simulink model "sampleModel1488"  (R2023a)
settings: Solver=VariableStepAuto  StartTime=0.0  StopTime=10.0  RelTol=1e-3
undefined symbols (not defined in the file): b011101a, b0c8, bf87616c, DiscIntNeverNeededParam, Newton, Raphson
libraries: simulink x171, slpidlib x32, simulink_need_slupdate x2
(part 3 of 6)

== system sampleModel1488/cfblk129/cfblk7 ==
  cfblk1 : Inport
  cfblk14 : Inport  Port=2
  cfblk15 : Inport  Port=3
  cfblk10 : Product  Inputs=**
  cfblk11 : Sum  Inputs=+-
  cfblk12 : Signum
  cfblk13 : Bias  Bias=[839960934.882999]  SaturateOnIntegerOverflow=off
  cfblk16 : Delay  SampleTime=1
  cfblk17 : Delay  SampleTime=1
  cfblk3 : slpidlib/PID Controller  Controller=PID  Form=Parallel  TimeDomain=Discrete-time  UseExternalTs=off  SampleTime=1  IntegratorMethod=Forward Euler  FilterMethod=Forward Euler  ControllerParametersSource=internal  P=1  I=1  UseKiTs=off  D=0  N=100  UseFilter=on  TunerSelectOption=Transfer Function Based (PID Tuner App)  InitialConditionSource=internal  InitialConditionForIntegrator=0  InitialConditionForFilter=0  DifferentiatorICPrevScaledInput=0  ExternalReset=none  TrackingMode=off  Kt=1  LimitOutput=off  SatLimitsSource=internal  UpperSaturationLimit=inf  LowerSaturationLimit=-inf  LinearizeAsGain=off  AntiWindupMode=none  Kb=1  LimitIntegrator=off  UpperIntegratorSaturationLimit=inf  LowerIntegratorSaturationLimit=-inf  POutMin=[]  POutMax=[]  IOutMin=[]  IOutMax=[]  DOutMin=[]  DOutMax=[]  NOutMin=[]  NOutMax=[]  SumOutMin=[]  SumOutMax=[]  SaturationOutMin=[]  SaturationOutMax=[]  PParamMin=[]  PParamMax=[]  IParamMin=[]  IParamMax=[]  DParamMin=[]  DParamMax=[]  NParamMin=[]  NParamMax=[]  KbParamMin=[]  KbParamMax=[]  KtParamMin=[]  KtParamMax=[]  KbOutMin=[]  KbOutMax=[]  KtOutMin=[]  KtOutMax=[]  IntegratorOutMin=[]  IntegratorOutMax=[]  FilterOutMin=[]  FilterOutMax=[]  SumI1OutMin=[]  SumI1OutMax=[]  SumI2OutMin=[]  SumI2OutMax=[]  SumI3OutMin=[]  SumI3OutMax=[]  SumI4OutMin=[]  SumI4OutMax=[]  SumDOutMin=[]  SumDOutMax=[]  DifferentiatorOutMin=[]  DifferentiatorOutMax=[]  FilterDiffOutCoefMin=[]  FilterDiffOutCoefMax=[]  ReciprocalOutMin=[]  ReciprocalOutMax=[]  SumDenOutMin=[]  SumDenOutMax=[]  SumNumOutMin=[]  SumNumOutMax=[]  DivideOutMin=[]  DivideOutMax=[]  UdiffTsProdOutMin=[]  UdiffTsProdOutMax=[]  NTsProdOutMin=[]  NTsProdOutMax=[]  UintegralTsProdOutMin=[]  UintegralTsProdOutMax=[]  UngainTsProdOutMin=[]  UngainTsProdOutMax=[]  ClampingZeroOutDataTypeStr=Inherit: Inherit via back propagation  ClampingZeroOutMin=[]  ClampingZeroOutMax=[]  FilterDenConstantOutDataTypeStr=Inherit: Inherit via back propagation  FilterDenConstantOutMin=[]  FilterDenConstantOutMax=[]  PCopyOutDataTypeStr=Inherit: Inherit via back propagation  PCopyOutMin=[]  PCopyOutMax=[]  NCopyOutDataTypeStr=Inherit: Inherit via back propagation  NCopyOutMin=[]  NCopyOutMax=[]  IntegratorContinuousStateAttributes=''  IntegratorStateMustResolveToSignalObject=off  IntegratorRTWStateStorageClass=Auto  FilterContinuousStateAttributes=''  FilterStateMustResolveToSignalObject=off  FilterRTWStateStorageClass=Auto  ParallelPVariant=InternalParameters  IdealPVariant=Disabled  IVariant=InternalParameters  DVariant=InternalParameters  IntegratorVariant=Discrete  SatVariant=Disabled  AWVariant=Passthrough  PCopyVariant=Disabled  TRVariant=Disabled  FdbkBlocksVariant=Forward  IdealPFdbkVariant=Disabled  SatFdbkVariant=Disabled  DerivativeFilterVariant=ForwardEulerFilter  NVariant=InternalParameters  NCopyVariant=Disabled  FilterICVariant=InternalICsFilter  IntegratorICVariant=InternalICs  ExternalResetVariant=Disabled  TRSumVariant=Passthrough  SumFdbkVariant=Disabled  SumVariant=Sum_PID  TsampFilterVariant=InternalTs  TsampNgainVariant=Passthrough  TsampIntegralVariant=Disabled_SignalSpec  ExternalSaturationOutDataTypeStr=Inherit: Same as second input
      settings: LibrarySourceBlock=simulink/Discrete/Discrete PID Controller
  cfblk4 : DiscreteFir  SampleTime=1
  cfblk5 : slpidlib/PID Controller  Controller=PID  Form=Parallel  TimeDomain=Discrete-time  UseExternalTs=off  SampleTime=1  IntegratorMethod=Forward Euler  FilterMethod=Forward Euler  ControllerParametersSource=internal  P=1  I=1  UseKiTs=off  D=0  N=100  UseFilter=on  TunerSelectOption=Transfer Function Based (PID Tuner App)  InitialConditionSource=internal  InitialConditionForIntegrator=0  InitialConditionForFilter=0  DifferentiatorICPrevScaledInput=0  ExternalReset=none  TrackingMode=off  Kt=1  LimitOutput=off  SatLimitsSource=internal  UpperSaturationLimit=inf  LowerSaturationLimit=-inf  LinearizeAsGain=off  AntiWindupMode=none  Kb=1  LimitIntegrator=off  UpperIntegratorSaturationLimit=inf  LowerIntegratorSaturationLimit=-inf  POutMin=[]  POutMax=[]  IOutMin=[]  IOutMax=[]  DOutMin=[]  DOutMax=[]  NOutMin=[]  NOutMax=[]  SumOutMin=[]  SumOutMax=[]  SaturationOutMin=[]  SaturationOutMax=[]  PParamMin=[]  PParamMax=[]  IParamMin=[]  IParamMax=[]  DParamMin=[]  DParamMax=[]  NParamMin=[]  NParamMax=[]  KbParamMin=[]  KbParamMax=[]  KtParamMin=[]  KtParamMax=[]  KbOutMin=[]  KbOutMax=[]  KtOutMin=[]  KtOutMax=[]  IntegratorOutMin=[]  IntegratorOutMax=[]  FilterOutMin=[]  FilterOutMax=[]  SumI1OutMin=[]  SumI1OutMax=[]  SumI2OutMin=[]  SumI2OutMax=[]  SumI3OutMin=[]  SumI3OutMax=[]  SumI4OutMin=[]  SumI4OutMax=[]  SumDOutMin=[]  SumDOutMax=[]  DifferentiatorOutMin=[]  DifferentiatorOutMax=[]  FilterDiffOutCoefMin=[]  FilterDiffOutCoefMax=[]  ReciprocalOutMin=[]  ReciprocalOutMax=[]  SumDenOutMin=[]  SumDenOutMax=[]  SumNumOutMin=[]  SumNumOutMax=[]  DivideOutMin=[]  DivideOutMax=[]  UdiffTsProdOutMin=[]  UdiffTsProdOutMax=[]  NTsProdOutMin=[]  NTsProdOutMax=[]  UintegralTsProdOutMin=[]  UintegralTsProdOutMax=[]  UngainTsProdOutMin=[]  UngainTsProdOutMax=[]  ClampingZeroOutDataTypeStr=Inherit: Inherit via back propagation  ClampingZeroOutMin=[]  ClampingZeroOutMax=[]  FilterDenConstantOutDataTypeStr=Inherit: Inherit via back propagation  FilterDenConstantOutMin=[]  FilterDenConstantOutMax=[]  PCopyOutDataTypeStr=Inherit: Inherit via back propagation  PCopyOutMin=[]  PCopyOutMax=[]  NCopyOutDataTypeStr=Inherit: Inherit via back propagation  NCopyOutMin=[]  NCopyOutMax=[]  IntegratorContinuousStateAttributes=''  IntegratorStateMustResolveToSignalObject=off  IntegratorRTWStateStorageClass=Auto  FilterContinuousStateAttributes=''  FilterStateMustResolveToSignalObject=off  FilterRTWStateStorageClass=Auto  ParallelPVariant=InternalParameters  IdealPVariant=Disabled  IVariant=InternalParameters  DVariant=InternalParameters  IntegratorVariant=Discrete  SatVariant=Disabled  AWVariant=Passthrough  PCopyVariant=Disabled  TRVariant=Disabled  FdbkBlocksVariant=Forward  IdealPFdbkVariant=Disabled  SatFdbkVariant=Disabled  DerivativeFilterVariant=ForwardEulerFilter  NVariant=InternalParameters  NCopyVariant=Disabled  FilterICVariant=InternalICsFilter  IntegratorICVariant=InternalICs  ExternalResetVariant=Disabled  TRSumVariant=Passthrough  SumFdbkVariant=Disabled  SumVariant=Sum_PID  TsampFilterVariant=InternalTs  TsampNgainVariant=Passthrough  TsampIntegralVariant=Disabled_SignalSpec  ExternalSaturationOutDataTypeStr=Inherit: Same as second input
      settings: LibrarySourceBlock=simulink/Discrete/Discrete PID Controller
  cfblk6 : simulink/Discrete/Difference  ICPrevInput=0.0  OutMin=[]  OutMax=[]  OutDataTypeStr=Inherit: Inherit via back propagation  OutDataType=fixdt(1, 16)  OutScaling=2^-10  DoSatur=off
  cfblk7 : slpidlib/PID Controller (2DOF)  Controller=PID  Form=Parallel  TimeDomain=Discrete-time  UseExternalTs=off  SampleTime=1  IntegratorMethod=Forward Euler  FilterMethod=Forward Euler  ControllerParametersSource=internal  P=1  I=1  UseKiTs=off  D=0  N=100  UseFilter=on  b=1  c=1  TunerSelectOption=Transfer Function Based (PID Tuner App)  InitialConditionSource=internal  InitialConditionForIntegrator=0  InitialConditionForFilter=0  DifferentiatorICPrevScaledInput=0  ExternalReset=none  TrackingMode=off  Kt=1  LimitOutput=off  SatLimitsSource=internal  UpperSaturationLimit=inf  LowerSaturationLimit=-inf  LinearizeAsGain=off  AntiWindupMode=none  Kb=1  LimitIntegrator=off  UpperIntegratorSaturationLimit=inf  LowerIntegratorSaturationLimit=-inf  POutMin=[]  POutMax=[]  IOutMin=[]  IOutMax=[]  DOutMin=[]  DOutMax=[]  NOutMin=[]  NOutMax=[]  bOutMin=[]  bOutMax=[]  cOutMin=[]  cOutMax=[]  SumOutMin=[]  SumOutMax=[]  SaturationOutMin=[]  SaturationOutMax=[]  PParamMin=[]  PParamMax=[]  IParamMin=[]  IParamMax=[]  DParamMin=[]  DParamMax=[]  NParamMin=[]  NParamMax=[]  bParamMin=[]  bParamMax=[]  cParamMin=[]  cParamMax=[]  KbParamMin=[]  KbParamMax=[]  KtParamMin=[]  KtParamMax=[]  KbOutMin=[]  KbOutMax=[]  KtOutMin=[]  KtOutMax=[]  IntegratorOutMin=[]  IntegratorOutMax=[]  FilterOutMin=[]  FilterOutMax=[]  SumI1OutMin=[]  SumI1OutMax=[]  SumI2OutMin=[]  SumI2OutMax=[]  SumI3OutMin=[]  SumI3OutMax=[]  SumI4OutMin=[]  SumI4OutMax=[]  SumDOutMin=[]  SumDOutMax=[]  Sum1OutMin=[]  Sum1OutMax=[]  Sum2OutMin=[]  Sum2OutMax=[]  Sum3OutMin=[]  Sum3OutMax=[]  DifferentiatorOutMin=[]  DifferentiatorOutMax=[]  FilterDiffOutCoefMin=[]  FilterDiffOutCoefMax=[]  ReciprocalOutMin=[]  ReciprocalOutMax=[]  SumDenOutMin=[]  SumDenOutMax=[]  SumNumOutMin=[]  SumNumOutMax=[]  DivideOutMin=[]  DivideOutMax=[]  UdiffTsProdOutMin=[]  UdiffTsProdOutMax=[]  NTsProdOutMin=[]  NTsProdOutMax=[]  UintegralTsProdOutMin=[]  UintegralTsProdOutMax=[]  UngainTsProdOutMin=[]  UngainTsProdOutMax=[]  ClampingZeroOutDataTypeStr=Inherit: Inherit via back propagation  ClampingZeroOutMin=[]  ClampingZeroOutMax=[]  FilterDenConstantOutDataTypeStr=Inherit: Inherit via back propagation  FilterDenConstantOutMin=[]  FilterDenConstantOutMax=[]  PCopyOutDataTypeStr=Inherit: Inherit via back propagation  PCopyOutMin=[]  PCopyOutMax=[]  NCopyOutDataTypeStr=Inherit: Inherit via back propagation  NCopyOutMin=[]  NCopyOutMax=[]  IntegratorContinuousStateAttributes=''  IntegratorStateMustResolveToSignalObject=off  IntegratorRTWStateStorageClass=Auto  FilterContinuousStateAttributes=''  FilterStateMustResolveToSignalObject=off  FilterRTWStateStorageClass=Auto  ParallelPVariant=InternalParameters  IdealPVariant=Disabled  IVariant=InternalParameters  DVariant=InternalParameters  bVariant=InternalParameters  cVariant=InternalParameters  IntegratorVariant=Discrete  SatVariant=Disabled  AWVariant=Passthrough  PCopyVariant=Disabled  TRVariant=Disabled  FdbkBlocksVariant=Forward  IdealPFdbkVariant=Disabled  SatFdbkVariant=Disabled  DerivativeFilterVariant=ForwardEulerFilter  NVariant=InternalParameters  NCopyVariant=Disabled  FilterICVariant=InternalICsFilter  IntegratorICVariant=InternalICs  ExternalResetVariant=Disabled  TRSumVariant=Passthrough  SumFdbkVariant=Disabled  SumVariant=Sum_PID  TsampFilterVariant=InternalTs  TsampNgainVariant=Passthrough  TsampIntegralVariant=Disabled_SignalSpec  ExternalSaturationOutDataTypeStr=Inherit: Same as second input
      settings: LibrarySourceBlock=simulink/Discrete/Discrete PID Controller (2DOF)
  cfblk8 : DiscreteFir  SampleTime=1
  cfblk9 : Sum  Inputs=|++
  cfblk2 : Outport
  wires:
  cfblk1/1 -> cfblk3/1
  cfblk3/1 -> cfblk5/1
  cfblk13/1 -> cfblk11/1
  cfblk9/1 -> cfblk2/1, cfblk10/2
  cfblk15/1 -> cfblk13/1, cfblk7/2
  cfblk4/1 -> cfblk7/1
  cfblk7/1 -> cfblk12/1
  cfblk8/1 -> cfblk6/1
  cfblk14/1 -> cfblk10/1
  cfblk10/1 -> cfblk8/1
  cfblk5/1 -> cfblk9/2
  cfblk6/1 -> cfblk11/2
  cfblk11/1 -> cfblk16/1
  cfblk16/1 -> cfblk9/1
  cfblk12/1 -> cfblk17/1
  cfblk17/1 -> cfblk4/1

== system sampleModel1488/cfblk129/cfblk8 ==
  cfblk1 : Inport
  cfblk8 : Inport  Port=2
  cfblk9 : Inport  Port=3
  cfblk3 : Delay  DelayLengthSource=Input port  SampleTime=1
      settings: InputPortMap=u0,p1
  cfblk4 : Sqrt  Operator=rSqrt  AlgorithmType=Newton-Raphson
  cfblk5 : Rounding
  cfblk6 : Rounding
  cfblk7 : Constant  Value=[787179622.880655]  SampleTime=1
  cfblk2 : Outport
  wires:
  cfblk5/1 -> cfblk6/1
  cfblk6/1 -> cfblk4/1
  cfblk9/1 -> cfblk3/1
  cfblk7/1 -> cfblk2/1
  cfblk8/1 -> cfblk5/1
  cfblk1/1 -> cfblk3/2

== system sampleModel1488/cfblk129/cfblk9 ==
  cfblk1 : Inport
  cfblk6 : Inport  Port=2
  cfblk7 : Inport  Port=3
  cfblk3 : simulink/Discrete/Transfer Fcn Lead or Lag  PoleZ=0.95  ZeroZ=0.75  ICPrevOutput=0.0  ICPrevInput=0.0  DoSatur=off
  cfblk4 : simulink/Discrete/Difference  ICPrevInput=0.0  OutMin=[]  OutMax=[]  OutDataTypeStr=Inherit: Inherit via back propagation  OutDataType=fixdt(1, 16)  OutScaling=2^-10  DoSatur=off
  cfblk5 : Signum
  cfblk2 : Outport
  wires:
  cfblk4/1 -> cfblk2/1
  cfblk1/1 -> cfblk4/1
  cfblk6/1 -> cfblk3/1
  cfblk7/1 -> cfblk5/1

== system sampleModel1488/cfblk130/cfblk10 ==
  cfblk1 : Inport
  cfblk8 : Inport  Port=2
  cfblk9 : Inport  Port=3
  cfblk10 : Inport  Port=4
  cfblk11 : Delay  SampleTime=1
  cfblk3 : simulink/Discrete/Transfer Fcn Lead or Lag  PoleZ=0.95  ZeroZ=0.75  ICPrevOutput=0.0  ICPrevInput=0.0  DoSatur=off
  cfblk4 : simulink/Discrete/Difference  ICPrevInput=0.0  OutMin=[]  OutMax=[]  OutDataTypeStr=Inherit: Inherit via back propagation  OutDataType=fixdt(1, 16)  OutScaling=2^-10  DoSatur=off
  cfblk5 : Product
  cfblk6 : Sum  Inputs=+-
  cfblk7 : Bias  Bias=[817095211.983372]  SaturateOnIntegerOverflow=off
  cfblk2 : Outport
  wires:
  cfblk7/1 -> cfblk6/1
  cfblk5/1 -> cfblk3/1
  cfblk9/1 -> cfblk2/1
  cfblk10/1 -> cfblk7/1
  cfblk1/1 -> cfblk5/1
  cfblk6/1 -> cfblk4/1
  cfblk8/1 -> cfblk6/2
  cfblk3/1 -> cfblk11/1
  cfblk11/1 -> cfblk5/2

== system sampleModel1488/cfblk130/cfblk7 ==
  cfblk1 : Inport
  cfblk10 : Inport  Port=2
  cfblk11 : Inport  Port=3
  cfblk12 : Inport  Port=4
  cfblk14 : Delay  SampleTime=1
  cfblk3 : DiscreteStateSpace
  cfblk4 : DiscreteStateSpace
  cfblk5 : Polyval  Coefs=[ +2.081618890e-019, -1.441693666e-014, +4.719686976e-010, -8.536869453e-006, +1.621573104e-001, -8.087801117e+001 ]
  cfblk6 : Product  Inputs=**
  cfblk7 : ComplexToMagnitudeAngle
  cfblk8 : Rounding
  cfblk9 : Constant  Value=[-610728300.679848]  SampleTime=1
  cfblk2 : Outport
  cfblk13 : Outport  Port=2
  wires:
  cfblk1/1 -> cfblk8/1
  cfblk3/1 -> cfblk13/1
  cfblk12/1 -> cfblk3/1
  cfblk7/1 -> cfblk6/1
  cfblk9/1 -> cfblk7/1
  cfblk4/1 -> cfblk5/1
  cfblk8/1 -> cfblk2/1
  cfblk7/2 -> cfblk6/2
  cfblk5/1 -> cfblk14/1
  cfblk14/1 -> cfblk4/1

== system sampleModel1488/cfblk130/cfblk8 ==
  cfblk1 : Inport
  cfblk10 : Inport  Port=2
  cfblk11 : Inport  Port=3
  cfblk3 : DiscreteFilter  SampleTime=1
  cfblk4 : DiscreteZeroPole  Poles=[0 0.5]  Gain=1
  cfblk5 : DiscreteTransferFcn  SampleTime=1
  cfblk6 : Product
  cfblk7 : Sin  TimeSource=Use external signal  SampleTime=0
  cfblk8 : Product
  cfblk9 : Constant  Value=[-842661004.303617]  SampleTime=1
  cfblk2 : Outport
  wires:
  cfblk3/1 -> cfblk2/1
  cfblk11/1 -> cfblk8/1
  cfblk7/1 -> cfblk8/2
  cfblk10/1 -> cfblk5/1
  cfblk9/1 -> cfblk3/1
  cfblk1/1 -> cfblk7/1
  cfblk6/1 -> cfblk4/1
  cfblk8/1 -> cfblk6/1
  cfblk5/1 -> cfblk6/2

== system sampleModel1488/cfblk130/cfblk9 ==
  cfblk1 : Inport
  cfblk12 : Inport  Port=2
  cfblk13 : Inport  Port=3
  cfblk10 : Sin  TimeSource=Use external signal  SampleTime=0
  cfblk11 : simulink/Math Operations/MinMax Running Resettable  Function=min  vinit=0.0
  cfblk16 : Delay  SampleTime=1
  cfblk17 : Delay  SampleTime=1
  cfblk3 : DiscreteTransferFcn  SampleTime=1
  cfblk4 : simulink/Discrete/Transfer Fcn Real Zero  ZeroZ=0.75  ICPrevInput=0.0  DoSatur=off
  cfblk5 : simulink/Math Operations/MinMax Running Resettable  Function=min  vinit=0.0
  cfblk6 : Abs  SaturateOnIntegerOverflow=off
  cfblk7 : Signum
  cfblk8 : Sum  Inputs=-+
  cfblk9 : Sum  Inputs=|++
  cfblk2 : Outport
  cfblk14 : Outport  Port=2
  cfblk15 : Outport  Port=3
  wires:
  cfblk1/1 -> cfblk5/1
  cfblk12/1 -> cfblk7/1
  cfblk10/1 -> cfblk2/1
  cfblk9/1 -> cfblk15/1
  cfblk6/1 -> cfblk8/1, cfblk9/2
  cfblk7/1 -> cfblk3/1, cfblk10/1
  cfblk11/1 -> cfblk4/1, cfblk16/1
  cfblk13/1 -> cfblk9/1, cfblk14/1
  cfblk3/1 -> cfblk6/1
  cfblk5/1 -> cfblk11/2
  cfblk4/1 -> cfblk8/2
  cfblk16/1 -> cfblk5/2
  cfblk8/1 -> cfblk17/1
  cfblk17/1 -> cfblk11/1

== system sampleModel1488/cfblk131/cfblk12 ==
  cfblk1 : Inport
  Action Port : ActionPort  ActionPortLabel=if(u1 >= 0)
  cfblk3 : Delay  ShowEnablePort=on
      settings: InputPortMap=u0,e6
  cfblk4 : Delay  DelayLengthSource=Input port
      settings: InputPortMap=u0,p1
  cfblk5 : MinMax  Function=max
  cfblk2 : Outport
  cfblk6 : Outport  Port=2
  cfblk7 : Outport  Port=3
  cfblk8 : Outport  Port=4
  wires:
  cfblk1/1 -> cfblk4/1, cfblk7/1, cfblk5/1, cfblk3/1, cfblk3/2
  cfblk4/1 -> cfblk2/1
  cfblk5/1 -> cfblk8/1, cfblk4/2
  cfblk3/1 -> cfblk6/1

== system sampleModel1488/cfblk131/cfblk13 ==
  cfblk1 : Inport
  cfblk9 : Inport  Port=2
  cfblk10 : Inport  Port=3
  Action Port : ActionPort  ActionPortLabel=else
  cfblk3 : ComplexToMagnitudeAngle
  cfblk4 : Sum  Inputs=-+
  cfblk5 : Squeeze
  cfblk6 : Signum
  cfblk7 : Squeeze
  cfblk8 : Sum  Inputs=|++
  cfblk2 : Outport
  cfblk11 : Outport  Port=2
  wires:
  cfblk7/1 -> cfblk6/1
  cfblk9/1 -> cfblk11/1
  cfblk5/1 -> cfblk7/1, cfblk4/2
  cfblk6/1 -> cfblk3/1
  cfblk8/1 -> cfblk2/1
  cfblk10/1 -> cfblk5/1
  cfblk1/1 -> cfblk4/1
  cfblk3/1 -> cfblk8/1
  cfblk3/2 -> cfblk8/2

== system sampleModel1488/cfblk131/cfblk8 ==
  cfblk1 : Inport
  cfblk16 : Inport  Port=2
  cfblk10 : simulink/Math Operations/Slider Gain  gain=1  low=0  high=2
  cfblk11 : Sum  Inputs=+
  cfblk12 : PermuteDimensions
  cfblk13 : simulink/Math Operations/MinMax Running Resettable  Function=min  vinit=0.0
  cfblk14 : Gain  Gain=[459161782.308450]
  cfblk15 : Constant  Value=[779212882.808627]  SampleTime=1
  cfblk17 : Delay  SampleTime=1
  cfblk3 : DiscreteIntegrator  ICPrevOutput=DiscIntNeverNeededParam  ICPrevScaledInput=DiscIntNeverNeededParam
  cfblk4 : DiscreteStateSpace
  cfblk5 : Rounding
  cfblk6 : Sum  Inputs=+-
  cfblk7 : Gain  Gain=[-468410068.072459]
  cfblk8 : Sin  TimeSource=Use external signal  SampleTime=0
  cfblk9 : Rounding
  cfblk2 : Outport
  wires:
  cfblk14/1 -> cfblk9/1
  cfblk1/1 -> cfblk10/1
  cfblk15/1 -> cfblk13/1
  cfblk11/1 -> cfblk12/1
  cfblk7/1 -> cfblk8/1
  cfblk8/1 -> cfblk6/1
  cfblk16/1 -> cfblk7/1
  cfblk3/1 -> cfblk5/1
  cfblk5/1 -> cfblk4/1
  cfblk9/1 -> cfblk2/1
  cfblk4/1 -> cfblk13/2
  cfblk13/1 -> cfblk6/2
  cfblk6/1 -> cfblk14/1
  cfblk10/1 -> cfblk3/1
  cfblk12/1 -> cfblk17/1
  cfblk17/1 -> cfblk11/1

== system sampleModel1488/cfblk131/cfblk9 ==
  cfblk1 : Inport
  cfblk10 : Rounding
  cfblk11 : Delay  SampleTime=1
  cfblk3 : DiscreteZeroPole  Poles=[0 0.5]  Gain=1
  cfblk4 : DiscreteIntegrator  ICPrevOutput=DiscIntNeverNeededParam  ICPrevScaledInput=DiscIntNeverNeededParam
  cfblk5 : simulink/Discrete/Transfer Fcn Lead or Lag  PoleZ=0.95  ZeroZ=0.75  ICPrevOutput=0.0  ICPrevInput=0.0  DoSatur=off
  cfblk6 : simulink/Discrete/Transfer Fcn Lead or Lag  PoleZ=0.95  ZeroZ=0.75  ICPrevOutput=0.0  ICPrevInput=0.0  DoSatur=off
  cfblk7 : Sum  Inputs=+-
  cfblk8 : Sum
  cfblk9 : Sin  TimeSource=Use external signal  SampleTime=0
  cfblk2 : Outport
  wires:
  cfblk4/1 -> cfblk2/1
  cfblk5/1 -> cfblk10/1
  cfblk8/1 -> cfblk3/1
  cfblk1/1 -> cfblk7/2
  cfblk10/1 -> cfblk9/1, cfblk8/2
  cfblk7/1 -> cfblk6/1, cfblk8/1
  cfblk6/1 -> cfblk5/1
  cfblk9/1 -> cfblk4/1
  cfblk3/1 -> cfblk11/1
  cfblk11/1 -> cfblk7/1

== system sampleModel1488/cfblk132/cfblk10 ==
  cfblk1 : Inport
  cfblk8 : Inport  Port=2
  cfblk9 : Inport  Port=3
  cfblk10 : Inport  Port=4
  cfblk11 : Inport  Port=5
  cfblk3 : UnitDelay  HasFrameUpgradeWarning=on
  cfblk4 : Abs  SaturateOnIntegerOverflow=off
  cfblk5 : DotProduct  OutDataTypeStr=Inherit: Inherit via internal rule
  cfblk6 : simulink/Math Operations/MinMax Running Resettable  Function=min  vinit=0.0
  cfblk7 : Constant  Value=[-259036778.791860]  SampleTime=1
  cfblk2 : Outport
  wires:
  cfblk3/1 -> cfblk6/1
  cfblk5/1 -> cfblk6/2
  cfblk7/1 -> cfblk4/1
  cfblk6/1 -> cfblk2/1
  cfblk11/1 -> cfblk3/1
  cfblk9/1 -> cfblk5/1
  cfblk1/1 -> cfblk5/2

== system sampleModel1488/cfblk132/cfblk11 ==
  cfblk1 : Inport
  cfblk12 : Inport  Port=2
  cfblk13 : Inport  Port=3
  cfblk14 : Inport  Port=4
  cfblk10 : Sum  Inputs=-+
  cfblk11 : Sin  TimeSource=Use external signal  SampleTime=0
  cfblk16 : Delay  SampleTime=1
  cfblk3 : slpidlib/PID Controller (2DOF)  Controller=PID  Form=Parallel  TimeDomain=Discrete-time  UseExternalTs=off  SampleTime=1  IntegratorMethod=Forward Euler  FilterMethod=Forward Euler  ControllerParametersSource=internal  P=1  I=1  UseKiTs=off  D=0  N=100  UseFilter=on  b=1  c=1  TunerSelectOption=Transfer Function Based (PID Tuner App)  InitialConditionSource=internal  InitialConditionForIntegrator=0  InitialConditionForFilter=0  DifferentiatorICPrevScaledInput=0  ExternalReset=none  TrackingMode=off  Kt=1  LimitOutput=off  SatLimitsSource=internal  UpperSaturationLimit=inf  LowerSaturationLimit=-inf  LinearizeAsGain=off  AntiWindupMode=none  Kb=1  LimitIntegrator=off  UpperIntegratorSaturationLimit=inf  LowerIntegratorSaturationLimit=-inf  POutMin=[]  POutMax=[]  IOutMin=[]  IOutMax=[]  DOutMin=[]  DOutMax=[]  NOutMin=[]  NOutMax=[]  bOutMin=[]  bOutMax=[]  cOutMin=[]  cOutMax=[]  SumOutMin=[]  SumOutMax=[]  SaturationOutMin=[]  SaturationOutMax=[]  PParamMin=[]  PParamMax=[]  IParamMin=[]  IParamMax=[]  DParamMin=[]  DParamMax=[]  NParamMin=[]  NParamMax=[]  bParamMin=[]  bParamMax=[]  cParamMin=[]  cParamMax=[]  KbParamMin=[]  KbParamMax=[]  KtParamMin=[]  KtParamMax=[]  KbOutMin=[]  KbOutMax=[]  KtOutMin=[]  KtOutMax=[]  IntegratorOutMin=[]  IntegratorOutMax=[]  FilterOutMin=[]  FilterOutMax=[]  SumI1OutMin=[]  SumI1OutMax=[]  SumI2OutMin=[]  SumI2OutMax=[]  SumI3OutMin=[]  SumI3OutMax=[]  SumI4OutMin=[]  SumI4OutMax=[]  SumDOutMin=[]  SumDOutMax=[]  Sum1OutMin=[]  Sum1OutMax=[]  Sum2OutMin=[]  Sum2OutMax=[]  Sum3OutMin=[]  Sum3OutMax=[]  DifferentiatorOutMin=[]  DifferentiatorOutMax=[]  FilterDiffOutCoefMin=[]  FilterDiffOutCoefMax=[]  ReciprocalOutMin=[]  ReciprocalOutMax=[]  SumDenOutMin=[]  SumDenOutMax=[]  SumNumOutMin=[]  SumNumOutMax=[]  DivideOutMin=[]  DivideOutMax=[]  UdiffTsProdOutMin=[]  UdiffTsProdOutMax=[]  NTsProdOutMin=[]  NTsProdOutMax=[]  UintegralTsProdOutMin=[]  UintegralTsProdOutMax=[]  UngainTsProdOutMin=[]  UngainTsProdOutMax=[]  ClampingZeroOutDataTypeStr=Inherit: Inherit via back propagation  ClampingZeroOutMin=[]  ClampingZeroOutMax=[]  FilterDenConstantOutDataTypeStr=Inherit: Inherit via back propagation  FilterDenConstantOutMin=[]  FilterDenConstantOutMax=[]  PCopyOutDataTypeStr=Inherit: Inherit via back propagation  PCopyOutMin=[]  PCopyOutMax=[]  NCopyOutDataTypeStr=Inherit: Inherit via back propagation  NCopyOutMin=[]  NCopyOutMax=[]  IntegratorContinuousStateAttributes=''  IntegratorStateMustResolveToSignalObject=off  IntegratorRTWStateStorageClass=Auto  FilterContinuousStateAttributes=''  FilterStateMustResolveToSignalObject=off  FilterRTWStateStorageClass=Auto  ParallelPVariant=InternalParameters  IdealPVariant=Disabled  IVariant=InternalParameters  DVariant=InternalParameters  bVariant=InternalParameters  cVariant=InternalParameters  IntegratorVariant=Discrete  SatVariant=Disabled  AWVariant=Passthrough  PCopyVariant=Disabled  TRVariant=Disabled  FdbkBlocksVariant=Forward  IdealPFdbkVariant=Disabled  SatFdbkVariant=Disabled  DerivativeFilterVariant=ForwardEulerFilter  NVariant=InternalParameters  NCopyVariant=Disabled  FilterICVariant=InternalICsFilter  IntegratorICVariant=InternalICs  ExternalResetVariant=Disabled  TRSumVariant=Passthrough  SumFdbkVariant=Disabled  SumVariant=Sum_PID  TsampFilterVariant=InternalTs  TsampNgainVariant=Passthrough  TsampIntegralVariant=Disabled_SignalSpec  ExternalSaturationOutDataTypeStr=Inherit: Same as second input
      settings: LibrarySourceBlock=simulink/Discrete/Discrete PID Controller (2DOF)
  cfblk4 : DiscreteStateSpace
  cfblk5 : simulink/Discrete/Tapped Delay  vinit=0.0  samptime=-1  NumDelays=1  DelayOrder=Oldest  includeCurrent=off
  cfblk6 : simulink/Discrete/Difference  ICPrevInput=0.0  OutMin=[]  OutMax=[]  OutDataTypeStr=Inherit: Inherit via back propagation  OutDataType=fixdt(1, 16)  OutScaling=2^-10  DoSatur=off
  cfblk7 : Sum  Inputs=|++
  cfblk8 : Sin  TimeSource=Use external signal  SampleTime=0
  cfblk9 : Signum
  cfblk2 : Outport
  cfblk15 : Outport  Port=2
  wires:
  cfblk3/1 -> cfblk5/1
  cfblk12/1 -> cfblk6/1
  cfblk11/1 -> cfblk3/1
  cfblk1/1 -> cfblk11/1
  cfblk14/1 -> cfblk3/2
  cfblk6/1 -> cfblk10/1
  cfblk4/1 -> cfblk15/1
  cfblk10/1 -> cfblk4/1, cfblk2/1
  cfblk5/1 -> cfblk7/1
  cfblk8/1 -> cfblk9/1
  cfblk13/1 -> cfblk7/2
  cfblk7/1 -> cfblk10/2
  cfblk9/1 -> cfblk16/1
  cfblk16/1 -> cfblk8/1

== system sampleModel1488/cfblk132/cfblk9 ==
  cfblk1 : Inport
  cfblk9 : Inport  Port=2
  cfblk10 : Inport  Port=3
  cfblk11 : Inport  Port=4
  cfblk3 : DiscreteStateSpace
  cfblk4 : Signum
  cfblk5 : Product
  cfblk6 : Signum
  cfblk7 : Constant  Value=[773930065.279327]  SampleTime=1
  cfblk8 : Constant  Value=[-380688371.941781]  SampleTime=1
  cfblk2 : Outport
  wires:
  cfblk8/1 -> cfblk6/1
  cfblk11/1 -> cfblk3/1
  cfblk1/1 -> cfblk5/1
  cfblk9/1 -> cfblk5/2
  cfblk7/1 -> cfblk2/1
  cfblk5/1 -> cfblk4/1

== system sampleModel1488/cfblk133/cfblk11 ==
  cfblk1 : Inport
  cfblk3 : ComplexToRealImag
  cfblk4 : Assignment  DiagnosticForDimensions=Warning  IndexOptions=Index vector (dialog)  Indices=1  OutputSizes=1
  cfblk5 : Gain  Gain=[641344015.890319]
  cfblk6 : Constant  Value=[-858026401.942738]  SampleTime=1
  cfblk8 : Delay  SampleTime=1
  cfblk2 : Outport
  cfblk7 : Outport  Port=2
  wires:
  cfblk4/1 -> cfblk5/1
  cfblk1/1 -> cfblk3/1
  cfblk3/1 -> cfblk7/1
  cfblk3/2 -> cfblk4/1
  cfblk6/1 -> cfblk2/1
  cfblk5/1 -> cfblk8/1
  cfblk8/1 -> cfblk4/2

== system sampleModel1488/cfblk133/cfblk12 ==
  cfblk1 : Inport
  cfblk3 : Delay  SampleTime=1
  cfblk4 : DiscreteFir  SampleTime=1
  cfblk5 : Sqrt
  cfblk6 : UnaryMinus
  cfblk7 : Sum  Inputs=|++
  cfblk8 : Constant  Value=[-605830765.974785]  SampleTime=1
  cfblk2 : Outport
  cfblk9 : Outport  Port=2
  cfblk10 : Outport  Port=3
  wires:
  cfblk7/1 -> cfblk4/1
  cfblk5/1 -> cfblk9/1
  cfblk4/1 -> cfblk3/1, cfblk5/1
  cfblk3/1 -> cfblk2/1
  cfblk8/1 -> cfblk6/1
  cfblk1/1 -> cfblk10/1, cfblk7/2
  cfblk6/1 -> cfblk7/1

== system sampleModel1488/cfblk133/cfblk13 ==
  cfblk1 : Inport
  cfblk8 : Inport  Port=2
  cfblk3 : DiscreteStateSpace
  cfblk4 : simulink/Math Operations/MinMax Running Resettable  Function=min  vinit=0.0
  cfblk5 : Sum  Inputs=+
  cfblk6 : PermuteDimensions
  cfblk7 : Constant  Value=[-192272514.252641]  SampleTime=1
  cfblk2 : Outport
  wires:
  cfblk1/1 -> cfblk6/1
  cfblk3/1 -> cfblk4/1
  cfblk6/1 -> cfblk3/1
  cfblk8/1 -> cfblk4/2
  cfblk4/1 -> cfblk2/1
  cfblk7/1 -> cfblk5/1

== system sampleModel1488/cfblk134/cfblk4 ==
  cfblk1 : Inport
  cfblk7 : Inport  Port=2
  cfblk8 : Inport  Port=3
  cfblk3 : Abs  SaturateOnIntegerOverflow=off
  cfblk4 : Sum  Inputs=+
  cfblk5 : Signum
  cfblk6 : Constant  Value=[913856729.958485]  SampleTime=1
  cfblk2 : Outport
  wires:
  cfblk3/1 -> cfblk5/1
  cfblk7/1 -> cfblk3/1
  cfblk5/1 -> cfblk2/1
  cfblk1/1 -> cfblk4/1

== system sampleModel1488/cfblk134/cfblk8 ==
  cfblk1 : Inport
  cfblk6 : Inport  Port=2
  Action Port : ActionPort  ActionPortLabel=if(u1 >= 0)
  cfblk3 : Sum  Inputs=|++
  cfblk4 : Math  Operator=10^u
  cfblk5 : Constant  Value=[241505950.785986]  SampleTime=1
  cfblk2 : Outport
  cfblk7 : Outport  Port=2
  wires:
  cfblk3/1 -> cfblk4/1
  cfblk4/1 -> cfblk7/1
  cfblk5/1 -> cfblk2/1
  cfblk1/1 -> cfblk3/1
  cfblk6/1 -> cfblk3/2

== system sampleModel1488/cfblk134/cfblk9 ==
  cfblk1 : Inport
  cfblk10 : Inport  Port=2
  cfblk11 : Inport  Port=3
  cfblk12 : Inport  Port=4
  Action Port : ActionPort  ActionPortLabel=else
  cfblk3 : simulink/Discrete/Transfer Fcn Lead or Lag  PoleZ=0.95  ZeroZ=0.75  ICPrevOutput=0.0  ICPrevInput=0.0  DoSatur=off
  cfblk4 : UnitDelay  SampleTime=-1  HasFrameUpgradeWarning=on
  cfblk5 : Delay
  cfblk6 : DiscreteZeroPole  Poles=[0 0.5]  Gain=1  SampleTime=-1
  cfblk7 : Product  Inputs=**
  cfblk8 : PermuteDimensions
  cfblk9 : Trigonometry
  cfblk2 : Outport
  cfblk13 : Outport  Port=2
  cfblk14 : Outport  Port=3
  cfblk15 : Outport  Port=4
  cfblk16 : Outport  Port=5
  wires:
  cfblk1/1 -> cfblk5/1
  cfblk10/1 -> cfblk4/1
  cfblk8/1 -> cfblk14/1
  cfblk12/1 -> cfblk7/1, cfblk13/1
  cfblk5/1 -> cfblk3/1
  cfblk11/1 -> cfblk7/2, cfblk15/1
  cfblk3/1 -> cfblk9/1
  cfblk4/1 -> cfblk2/1
  cfblk9/1 -> cfblk8/1
  cfblk6/1 -> cfblk16/1
  cfblk7/1 -> cfblk6/1

== system sampleModel1488/cfblk135/cfblk12 ==
  cfblk1 : Inport
  cfblk7 : Inport  Port=2
  cfblk8 : Inport  Port=3
  cfblk9 : Inport  Port=4
  cfblk11 : Delay  SampleTime=1
  cfblk3 : PropagationDelay  SampleTime=1
  cfblk4 : simulink/Discrete/Difference  ICPrevInput=0.0  OutMin=[]  OutMax=[]  OutDataTypeStr=Inherit: Inherit via back propagation  OutDataType=fixdt(1, 16)  OutScaling=2^-10  DoSatur=off
  cfblk5 : Product  Inputs=**
  cfblk6 : Trigonometry
  cfblk2 : Outport
  cfblk10 : Outport  Port=2
  wires:
  cfblk7/1 -> cfblk3/1
  cfblk4/1 -> cfblk10/1
  cfblk9/1 -> cfblk4/1
  cfblk8/1 -> cfblk2/1
  cfblk6/1 -> cfblk5/1
  cfblk1/1 -> cfblk6/1
  cfblk5/1 -> cfblk3/2
  cfblk3/1 -> cfblk11/1
  cfblk11/1 -> cfblk5/2

== system sampleModel1488/cfblk135/cfblk13 ==
  cfblk1 : Inport
  cfblk6 : Inport  Port=2
  cfblk7 : Inport  Port=3
  cfblk3 : PropagationDelay  SampleTime=1
  cfblk4 : DiscreteIntegrator  ICPrevOutput=DiscIntNeverNeededParam  ICPrevScaledInput=DiscIntNeverNeededParam
  cfblk5 : Rounding
  cfblk2 : Outport
  cfblk8 : Outport  Port=2
  wires:
  cfblk4/1 -> cfblk3/1
  cfblk3/1 -> cfblk2/1
  cfblk1/1 -> cfblk5/1
  cfblk7/1 -> cfblk4/1
  cfblk6/1 -> cfblk3/2
  cfblk5/1 -> cfblk8/1

== system sampleModel1488/cfblk135/cfblk14 ==
  cfblk1 : Inport
  cfblk14 : Inport  Port=2
  cfblk15 : Inport  Port=3
  cfblk16 : Inport  Port=4
  cfblk10 : Sum  Inputs=+
  cfblk11 : Product
  cfblk12 : Constant  Value=[-278172261.717273]  SampleTime=1
  cfblk13 : Constant  Value=[-589429660.723729]  SampleTime=1
  cfblk3 : DiscreteIntegrator  ICPrevOutput=DiscIntNeverNeededParam  ICPrevScaledInput=DiscIntNeverNeededParam
  cfblk4 : Polyval  Coefs=[ +2.081618890e-019, -1.441693666e-014, +4.719686976e-010, -8.536869453e-006, +1.621573104e-001, -8.087801117e+001 ]
  cfblk5 : Sum  Inputs=|++
  cfblk6 : Reshape
  cfblk7 : Sum  Inputs=-+
  cfblk8 : Math  Operator=10^u
  cfblk9 : Bias  Bias=[-877762042.695378]  SaturateOnIntegerOverflow=off
  cfblk2 : Outport
  cfblk17 : Outport  Port=2
  wires:
  cfblk16/1 -> cfblk6/1
  cfblk3/1 -> cfblk11/1
  cfblk13/1 -> cfblk10/1
  cfblk10/1 -> cfblk5/1
  cfblk15/1 -> cfblk8/1
  cfblk14/1 -> cfblk3/1
  cfblk4/1 -> cfblk7/1
  cfblk6/1 -> cfblk11/2
  cfblk11/1 -> cfblk2/1
  cfblk9/1 -> cfblk4/1
  cfblk1/1 -> cfblk9/1
  cfblk12/1 -> cfblk7/2
  cfblk7/1 -> cfblk5/2
  cfblk5/1 -> cfblk17/1

== system sampleModel1488/cfblk135/cfblk15 ==
  cfblk1 : Inport
  cfblk14 : Inport  Port=2
  cfblk15 : Inport  Port=3
  cfblk10 : Constant  Value=[-619212913.210201]  SampleTime=1
  cfblk11 : Constant  Value=[-559190623.228161]  SampleTime=1
  cfblk12 : Constant  Value=[203635179.405806]  SampleTime=1
  cfblk13 : Constant  Value=[-264079852.924604]  SampleTime=1
  cfblk3 : DiscreteZeroPole  Poles=[0 0.5]  Gain=1
  cfblk4 : Delay  DelayLengthSource=Input port  SampleTime=1
      settings: InputPortMap=u0,p1
  cfblk5 : Signum
  cfblk6 : ComplexToMagnitudeAngle
  cfblk7 : Sum  Inputs=+-
  cfblk8 : simulink/Math Operations/Slider Gain  gain=1  low=0  high=2
  cfblk9 : Squeeze
  cfblk2 : Outport
  cfblk16 : Outport  Port=2
  wires:
  cfblk4/1 -> cfblk2/1
  cfblk12/1 -> cfblk3/1
  cfblk10/1 -> cfblk7/1
  cfblk1/1 -> cfblk5/1
  cfblk6/1 -> cfblk4/1
  cfblk3/1 -> cfblk8/1
  cfblk7/1 -> cfblk4/2
  cfblk8/1 -> cfblk7/2
  cfblk13/1 -> cfblk9/1
  cfblk14/1 -> cfblk16/1
  cfblk5/1 -> cfblk6/1

== system sampleModel1488/cfblk136/cfblk9 ==
  cfblk1 : Inport
  cfblk9 : Inport  Port=2
  cfblk10 : Inport  Port=3
  cfblk3 : simulink/Discrete/Difference  ICPrevInput=0.0  OutMin=[]  OutMax=[]  OutDataTypeStr=Inherit: Inherit via back propagation  OutDataType=fixdt(1, 16)  OutScaling=2^-10  DoSatur=off
  cfblk4 : simulink/Discrete/Difference  ICPrevInput=0.0  OutMin=[]  OutMax=[]  OutDataTypeStr=Inherit: Inherit via back propagation  OutDataType=fixdt(1, 16)  OutScaling=2^-10  DoSatur=off
  cfblk5 : Sum  Inputs=+
  cfblk6 : Gain  Gain=[-166635587.038039]
  cfblk7 : Rounding
  cfblk8 : Constant  Value=[-185283362.667530]  SampleTime=1
  cfblk2 : Outport
  cfblk11 : Outport  Port=2
  wires:
  cfblk9/1 -> cfblk5/1
  cfblk5/1 -> cfblk4/1
  cfblk8/1 -> cfblk6/1
  cfblk7/1 -> cfblk3/1
  cfblk3/1 -> cfblk11/1
  cfblk4/1 -> cfblk2/1
  cfblk6/1 -> cfblk7/1

== system sampleModel1488/cfblk137/cfblk13 ==
  cfblk1 : Inport
  cfblk10 : Inport  Port=2
  cfblk11 : Inport  Port=3
  cfblk12 : Inport  Port=4
  cfblk3 : simulink/Discrete/Tapped Delay  vinit=0.0  samptime=-1  NumDelays=1  DelayOrder=Oldest  includeCurrent=off
  cfblk4 : simulink/Math Operations/Slider Gain  gain=1  low=0  high=2
  cfblk5 : Abs  SaturateOnIntegerOverflow=off
  cfblk6 : Product
  cfblk7 : UnaryMinus
  cfblk8 : Constant  Value=[-190552281.993715]  SampleTime=1
  cfblk9 : Constant  Value=[-914391506.724116]  SampleTime=1
  cfblk2 : Outport
  cfblk13 : Outport  Port=2
  wires:
  cfblk9/1 -> cfblk7/1
  cfblk7/1 -> cfblk6/1
  cfblk1/1 -> cfblk4/1
  cfblk4/1 -> cfblk6/2
  cfblk6/1 -> cfblk2/1
  cfblk12/1 -> cfblk3/1
  cfblk11/1 -> cfblk5/1
  cfblk8/1 -> cfblk13/1

== system sampleModel1488/cfblk137/cfblk14 ==
  cfblk1 : Inport
  cfblk10 : Inport  Port=2
  cfblk11 : Inport  Port=3
  cfblk12 : Inport  Port=4
  cfblk15 : Delay  SampleTime=1
  cfblk3 : simulink/Discrete/Transfer Fcn Real Zero  ZeroZ=0.75  ICPrevInput=0.0  DoSatur=off
  cfblk4 : Delay  SampleTime=1
  cfblk5 : simulink/Discrete/Transfer Fcn First Order  PoleZ=0.95  ICPrevOutput=0.0  DoSatur=off
  cfblk6 : Delay  DelayLengthSource=Input port  SampleTime=1
      settings: InputPortMap=u0,p1
  cfblk7 : Signum
  cfblk8 : Signum
  cfblk9 : ComplexToRealImag
  cfblk2 : Outport
  cfblk13 : Outport  Port=2
  cfblk14 : Outport  Port=3
  wires:
  cfblk4/1 -> cfblk7/1
  cfblk11/1 -> cfblk8/1
  cfblk12/1 -> cfblk9/1
  cfblk3/1 -> cfblk13/1
  cfblk8/1 -> cfblk3/1
  cfblk1/1 -> cfblk4/1
  cfblk7/1 -> cfblk14/1
  cfblk10/1 -> cfblk2/1
  cfblk5/1 -> cfblk6/1
  cfblk9/1 -> cfblk6/2
  cfblk6/1 -> cfblk15/1
  cfblk15/1 -> cfblk5/1

== system sampleModel1488/cfblk137/cfblk15 ==
  cfblk1 : Inport
  cfblk8 : Inport  Port=2
  cfblk9 : Inport  Port=3
  cfblk10 : Inport  Port=4
  cfblk3 : DiscreteStateSpace
  cfblk4 : ComplexToRealImag
  cfblk5 : Sin  TimeSource=Use external signal  SampleTime=0
  cfblk6 : Trigonometry
  cfblk7 : Constant  Value=[-603946704.757632]  SampleTime=1
  cfblk2 : Outport
  cfblk11 : Outport  Port=2
  wires:
  cfblk8/1 -> cfblk5/1
  cfblk7/1 -> cfblk4/1
  cfblk9/1 -> cfblk11/1
  cfblk10/1 -> cfblk2/1
  cfblk5/1 -> cfblk6/1
  cfblk1/1 -> cfblk3/1

== system sampleModel1488/cfblk138/cfblk7 ==
  cfblk1 : Inport
  cfblk5 : Inport  Port=2
  cfblk6 : Inport  Port=3
  cfblk3 : simulink/Discrete/Transfer Fcn Lead or Lag  PoleZ=0.95  ZeroZ=0.75  ICPrevOutput=0.0  ICPrevInput=0.0  DoSatur=off
  cfblk4 : DotProduct  OutDataTypeStr=Inherit: Inherit via internal rule
  cfblk8 : Delay  SampleTime=1
  cfblk2 : Outport
  cfblk7 : Outport  Port=2
  wires:
  cfblk6/1 -> cfblk7/1
  cfblk1/1 -> cfblk4/2
  cfblk5/1 -> cfblk2/1
  cfblk4/1 -> cfblk3/1
  cfblk3/1 -> cfblk8/1
  cfblk8/1 -> cfblk4/1

== system sampleModel1488/cfblk138/cfblk8 ==
  cfblk1 : Inport
  cfblk9 : Inport  Port=2
  cfblk3 : simulink/Discrete/Transfer Fcn First Order  PoleZ=0.95  ICPrevOutput=0.0  DoSatur=off
  cfblk4 : DiscreteZeroPole  Poles=[0 0.5]  Gain=1
  cfblk5 : UnaryMinus
  cfblk6 : Math
  cfblk7 : UnaryMinus
  cfblk8 : Sum  Inputs=+
  cfblk2 : Outport
  cfblk10 : Outport  Port=2
  wires:
  cfblk4/1 -> cfblk6/1
  cfblk8/1 -> cfblk10/1
  cfblk6/1 -> cfblk7/1
  cfblk3/1 -> cfblk2/1
  cfblk5/1 -> cfblk4/1
  cfblk9/1 -> cfblk5/1
  cfblk1/1 -> cfblk8/1
  cfblk7/1 -> cfblk3/1

== system sampleModel1488/cfblk139/cfblk10 ==
  cfblk1 : Inport
  cfblk8 : Inport  Port=2
  cfblk3 : Delay  SampleTime=1
  cfblk4 : Delay  ShowEnablePort=on  SampleTime=1
      settings: InputPortMap=u0,e6
  cfblk5 : Reshape
  cfblk6 : Product  Inputs=**
  cfblk7 : Constant  Value=[-617109439.617472]  SampleTime=1
  cfblk2 : Outport
  wires:
  cfblk8/1 -> cfblk4/1
  cfblk5/1 -> cfblk4/2
  cfblk7/1 -> cfblk3/1
  cfblk1/1 -> cfblk5/1, cfblk6/2
  cfblk4/1 -> cfblk2/1
  cfblk3/1 -> cfblk6/1

== system sampleModel1488/cfblk139/cfblk11 ==
  cfblk1 : Inport
  cfblk7 : Inport  Port=2
  cfblk8 : Inport  Port=3
  cfblk9 : Inport  Port=4
  cfblk11 : Delay  SampleTime=1
  cfblk3 : DiscreteStateSpace
  cfblk4 : Math  Operator=rem
  cfblk5 : Assignment  DiagnosticForDimensions=Warning  IndexOptions=Index vector (dialog)  Indices=1  OutputSizes=1
  cfblk6 : Reshape
  cfblk2 : Outport
  cfblk10 : Outport  Port=2
  wires:
  cfblk9/1 -> cfblk2/1
  cfblk7/1 -> cfblk6/1
  cfblk1/1 -> cfblk4/2
  cfblk8/1 -> cfblk3/1
  cfblk3/1 -> cfblk5/1
  cfblk4/1 -> cfblk5/2
  cfblk6/1 -> cfblk10/1
  cfblk5/1 -> cfblk11/1
  cfblk11/1 -> cfblk4/1

== system sampleModel1488/cfblk139/cfblk12 ==
  cfblk1 : Inport
  cfblk7 : Inport  Port=2
  cfblk8 : Inport  Port=3
  cfblk9 : Inport  Port=4
  cfblk10 : Inport  Port=5
  cfblk11 : Delay  SampleTime=1
  cfblk3 : DiscreteIntegrator  ICPrevOutput=DiscIntNeverNeededParam  ICPrevScaledInput=DiscIntNeverNeededParam
  cfblk4 : DiscreteIntegrator  ICPrevOutput=DiscIntNeverNeededParam  ICPrevScaledInput=DiscIntNeverNeededParam
  cfblk5 : simulink/Math Operations/MinMax Running Resettable  Function=min  vinit=0.0
  cfblk6 : Constant  Value=[159069157.716894]  SampleTime=1
  cfblk2 : Outport
  wires:
  cfblk9/1 -> cfblk3/1
  cfblk7/1 -> cfblk2/1
  cfblk10/1 -> cfblk5/1
  cfblk4/1 -> cfblk5/2
  cfblk5/1 -> cfblk11/1
  cfblk11/1 -> cfblk4/1

== system sampleModel1488/cfblk139/cfblk8 ==
  cfblk1 : Inport
  cfblk5 : Inport  Port=2
  cfblk3 : DiscreteFilter  SampleTime=1
  cfblk4 : Math  Operator=log
  cfblk2 : Outport
  cfblk6 : Outport  Port=2
  cfblk7 : Outport  Port=3
  wires:
  cfblk1/1 -> cfblk6/1, cfblk3/1
  cfblk5/1 -> cfblk7/1
  cfblk3/1 -> cfblk4/1
  cfblk4/1 -> cfblk2/1

== system sampleModel1488/cfblk139/cfblk9 ==
  cfblk1 : Inport
  cfblk13 : Inport  Port=2
  cfblk14 : Inport  Port=3
  cfblk15 : Inport  Port=4
  cfblk10 : Squeeze
  cfblk11 : Product  Inputs=**
  cfblk12 : Constant  Value=[991796350.161302]  SampleTime=1
  cfblk3 : simulink/Discrete/Transfer Fcn First Order  PoleZ=0.95  ICPrevOutput=0.0  DoSatur=off
  cfblk4 : DiscreteZeroPole  Poles=[0 0.5]  Gain=1
  cfblk5 : DiscreteIntegrator  ICPrevOutput=DiscIntNeverNeededParam  ICPrevScaledInput=DiscIntNeverNeededParam
  cfblk6 : Delay  DelayLengthSource=Input port  SampleTime=1
      settings: InputPortMap=u0,p1
  cfblk7 : UnaryMinus
  cfblk8 : Abs  SaturateOnIntegerOverflow=off
  cfblk9 : Sum  Inputs=+-
  cfblk2 : Outport
  cfblk16 : Outport  Port=2
  wires:
  cfblk5/1 -> cfblk8/1
  cfblk1/1 -> cfblk10/1
  cfblk12/1 -> cfblk3/1
  cfblk13/1 -> cfblk4/1
  cfblk4/1 -> cfblk7/1
  cfblk14/1 -> cfblk11/1
  cfblk10/1 -> cfblk11/2
  cfblk8/1 -> cfblk9/1
  cfblk15/1 -> cfblk5/1
  cfblk7/1 -> cfblk6/1
  cfblk6/1 -> cfblk2/1
  cfblk9/1 -> cfblk16/1
  cfblk11/1 -> cfblk6/2
  cfblk3/1 -> cfblk9/2

== system sampleModel1488/cfblk140/cfblk7 ==
  cfblk1 : Inport
  cfblk11 : Inport  Port=2
  cfblk12 : Inport  Port=3
  cfblk10 : Constant  Value=[687991863.977745]  SampleTime=1
  cfblk3 : DiscreteStateSpace
  cfblk4 : simulink/Discrete/Transfer Fcn Lead or Lag  PoleZ=0.95  ZeroZ=0.75  ICPrevOutput=0.0  ICPrevInput=0.0  DoSatur=off
  cfblk5 : DiscreteZeroPole  Poles=[0 0.5]  Gain=1
  cfblk6 : simulink/Discrete/Transfer Fcn Lead or Lag  PoleZ=0.95  ZeroZ=0.75  ICPrevOutput=0.0  ICPrevInput=0.0  DoSatur=off
  cfblk7 : simulink/Discrete/Difference  ICPrevInput=0.0  OutMin=[]  OutMax=[]  OutDataTypeStr=Inherit: Inherit via back propagation  OutDataType=fixdt(1, 16)  OutScaling=2^-10  DoSatur=off
  cfblk8 : DiscreteTransferFcn  SampleTime=1
  cfblk9 : Polyval  Coefs=[ +2.081618890e-019, -1.441693666e-014, +4.719686976e-010, -8.536869453e-006, +1.621573104e-001, -8.087801117e+001 ]
  cfblk2 : Outport
  cfblk13 : Outport  Port=2
  cfblk14 : Outport  Port=3
  wires:
  cfblk11/1 -> cfblk7/1
  cfblk3/1 -> cfblk2/1
  cfblk7/1 -> cfblk4/1
  cfblk1/1 -> cfblk9/1
  cfblk6/1 -> cfblk5/1
  cfblk8/1 -> cfblk6/1
  cfblk9/1 -> cfblk14/1
  cfblk10/1 -> cfblk13/1
  cfblk5/1 -> cfblk3/1
  cfblk4/1 -> cfblk8/1

== system sampleModel1488/cfblk140/cfblk8 ==
  cfblk1 : Inport
  cfblk10 : Inport  Port=2
  cfblk12 : Delay  SampleTime=1
  cfblk3 : DiscreteStateSpace
  cfblk4 : DiscreteZeroPole  Poles=[0 0.5]  Gain=1
  cfblk5 : PermuteDimensions
  cfblk6 : Assignment  DiagnosticForDimensions=Warning  IndexOptions=Index vector (dialog)  Indices=1  OutputSizes=1
  cfblk7 : UnaryMinus
  cfblk8 : Sum  Inputs=+
  cfblk9 : Constant  Value=[986904709.045283]  SampleTime=1
  cfblk2 : Outport
  cfblk11 : Outport  Port=2
  wires:
  cfblk3/1 -> cfblk6/1
  cfblk6/1 -> cfblk5/1
  cfblk1/1 -> cfblk2/1
  cfblk5/1 -> cfblk11/1
  cfblk4/1 -> cfblk3/1
  cfblk9/1 -> cfblk4/1
  cfblk10/1 -> cfblk6/2
  cfblk7/1 -> cfblk8/1
  cfblk8/1 -> cfblk12/1
  cfblk12/1 -> cfblk7/1

== system sampleModel1488/cfblk141/cfblk10 ==
  cfblk1 : Inport
  cfblk3 : DiscreteFilter  SampleTime=1
  cfblk4 : Polyval  Coefs=[ +2.081618890e-019, -1.441693666e-014, +4.719686976e-010, -8.536869453e-006, +1.621573104e-001, -8.087801117e+001 ]
  cfblk5 : simulink/Math Operations/MinMax Running Resettable  Function=min  vinit=0.0
  cfblk6 : Constant  Value=[-199239202.035362]  SampleTime=1
  cfblk7 : Constant  Value=[83399863.738537]  SampleTime=1
  cfblk8 : Delay  SampleTime=1
  cfblk2 : Outport
  wires:
  cfblk3/1 -> cfblk2/1
  cfblk7/1 -> cfblk5/1
  cfblk6/1 -> cfblk3/1
  cfblk4/1 -> cfblk5/2
  cfblk5/1 -> cfblk8/1
  cfblk8/1 -> cfblk4/1

== system sampleModel1488/cfblk141/cfblk11 ==
  cfblk1 : Inport
  cfblk6 : Inport  Port=2
  cfblk3 : PermuteDimensions
  cfblk4 : Sqrt  Operator=rSqrt  AlgorithmType=Newton-Raphson
  cfblk5 : Constant  Value=[228980796.522772]  SampleTime=1
  cfblk2 : Outport
  cfblk7 : Outport  Port=2
  wires:
  cfblk4/1 -> cfblk7/1
  cfblk3/1 -> cfblk4/1
  cfblk1/1 -> cfblk2/1
  cfblk6/1 -> cfblk3/1

== system sampleModel1488/cfblk141/cfblk9 ==
  cfblk1 : Inport
  cfblk7 : Inport  Port=2
  cfblk8 : Inport  Port=3
  cfblk9 : Inport  Port=4
  cfblk3 : simulink/Discrete/Transfer Fcn Lead or Lag  PoleZ=0.95  ZeroZ=0.75  ICPrevOutput=0.0  ICPrevInput=0.0  DoSatur=off
  cfblk4 : MinMax  Function=max
  cfblk5 : Math  Operator=10^u
  cfblk6 : Constant  Value=[822693086.321830]  SampleTime=1
  cfblk2 : Outport
  cfblk10 : Outport  Port=2
  cfblk11 : Outport  Port=3
  wires:
  cfblk3/1 -> cfblk11/1
  cfblk7/1 -> cfblk5/1
  cfblk8/1 -> cfblk10/1
  cfblk9/1 -> cfblk2/1
  cfblk6/1 -> cfblk4/1
  cfblk5/1 -> cfblk3/1

== system sampleModel1488/cfblk142/cfblk4 ==
  cfblk1 : Inport
  cfblk13 : Inport  Port=2
  cfblk14 : Inport  Port=3
  cfblk10 : Reshape
  cfblk11 : Constant  Value=[698451375.296782]  SampleTime=1
  cfblk12 : Constant  Value=[429920940.729578]  SampleTime=1
  cfblk3 : DiscreteFilter  SampleTime=1
  cfblk4 : DiscreteIntegrator  ICPrevOutput=DiscIntNeverNeededParam  ICPrevScaledInput=DiscIntNeverNeededParam
  cfblk5 : DiscreteTransferFcn  SampleTime=1
  cfblk6 : DiscreteFilter  SampleTime=1
  cfblk7 : simulink/Discrete/Transfer Fcn First Order  PoleZ=0.95  ICPrevOutput=0.0  DoSatur=off
  cfblk8 : UnaryMinus
  cfblk9 : Math  Operator=10^u
  cfblk2 : Outport
  cfblk15 : Outport  Port=2
  wires:
  cfblk11/1 -> cfblk6/1
  cfblk1/1 -> cfblk15/1
  cfblk9/1 -> cfblk4/1
  cfblk5/1 -> cfblk2/1
  cfblk6/1 -> cfblk8/1
  cfblk7/1 -> cfblk9/1
  cfblk3/1 -> cfblk10/1
  cfblk8/1 -> cfblk3/1
  cfblk10/1 -> cfblk7/1
  cfblk4/1 -> cfblk5/1

== system sampleModel1488/cfblk142/cfblk5 ==
  cfblk1 : Inport
  cfblk6 : Inport  Port=2
  cfblk7 : Inport  Port=3
  cfblk3 : Product
  cfblk4 : Product  Inputs=**
  cfblk5 : Constant  Value=[670870212.898370]  SampleTime=1
  cfblk2 : Outport
  cfblk8 : Outport  Port=2
  wires:
  cfblk4/1 -> cfblk2/1
  cfblk3/1 -> cfblk4/1
  cfblk7/1 -> cfblk8/1
  cfblk5/1 -> cfblk3/1
  cfblk1/1 -> cfblk4/2
  cfblk6/1 -> cfblk3/2

== system sampleModel1488/cfblk142/cfblk6 ==
  cfblk1 : Inport
  cfblk12 : Inport  Port=2
  cfblk13 : Inport  Port=3
  cfblk14 : Inport  Port=4
  cfblk15 : Inport  Port=5
  cfblk16 : Inport  Port=6
  cfblk10 : simulink/Math Operations/MinMax Running Resettable  Function=min  vinit=0.0
  cfblk11 : Constant  Value=[-288878495.062511]  SampleTime=1
  cfblk18 : Delay  SampleTime=1
  cfblk3 : Delay  SampleTime=1
  cfblk4 : simulink/Discrete/Transfer Fcn First Order  PoleZ=0.95  ICPrevOutput=0.0  DoSatur=off
  cfblk5 : PropagationDelay  SampleTime=1
  cfblk6 : UnitDelay  HasFrameUpgradeWarning=on
  cfblk7 : simulink/Math Operations/MinMax Running Resettable  Function=min  vinit=0.0
  cfblk8 : simulink/Math Operations/MinMax Running Resettable  Function=min  vinit=0.0
  cfblk9 : UnaryMinus
  cfblk2 : Outport
  cfblk17 : Outport  Port=2
  wires:
  cfblk11/1 -> cfblk10/1
  cfblk8/1 -> cfblk7/1
  cfblk14/1 -> cfblk4/1
  cfblk6/1 -> cfblk9/1
  cfblk13/1 -> cfblk2/1
  cfblk5/1 -> cfblk6/1
  cfblk16/1 -> cfblk10/2
  cfblk10/1 -> cfblk7/2
  cfblk12/1 -> cfblk8/1
  cfblk9/1 -> cfblk8/2
  cfblk3/1 -> cfblk17/1
  cfblk1/1 -> cfblk3/1
  cfblk15/1 -> cfblk5/2
  cfblk7/1 -> cfblk18/1
  cfblk18/1 -> cfblk5/1

== system sampleModel1488/cfblk142/cfblk7 ==
  cfblk1 : Inport
  cfblk10 : Rounding
  cfblk11 : Product
  cfblk12 : Sqrt  Operator=rSqrt  AlgorithmType=Newton-Raphson
  cfblk13 : Constant  Value=[-91957907.379746]  SampleTime=1
  cfblk14 : Constant  Value=[-330454925.062983]  SampleTime=1
  cfblk3 : simulink/Discrete/Tapped Delay  vinit=0.0  samptime=-1  NumDelays=1  DelayOrder=Oldest  includeCurrent=off
  cfblk4 : DiscreteStateSpace
  cfblk5 : UnitDelay  HasFrameUpgradeWarning=on
  cfblk6 : Delay  SampleTime=1
  cfblk7 : Polyval  Coefs=[ +2.081618890e-019, -1.441693666e-014, +4.719686976e-010, -8.536869453e-006, +1.621573104e-001, -8.087801117e+001 ]
  cfblk8 : Sum  Inputs=+
  cfblk9 : Sum  Inputs=-+
  cfblk2 : Outport
  cfblk15 : Outport  Port=2
  wires:
  cfblk4/1 -> cfblk7/1
  cfblk1/1 -> cfblk6/1
  cfblk5/1 -> cfblk15/1
  cfblk8/1 -> cfblk12/1
  cfblk9/1 -> cfblk3/1
  cfblk11/1 -> cfblk9/1
  cfblk12/1 -> cfblk5/1
  cfblk13/1 -> cfblk4/1
  cfblk6/1 -> cfblk2/1
  cfblk10/1 -> cfblk11/1
  cfblk14/1 -> cfblk9/2
  cfblk7/1 -> cfblk11/2, cfblk10/1
  cfblk3/1 -> cfblk8/1

== system sampleModel1488/cfblk143/cfblk10 ==
  cfblk1 : Inport
  cfblk7 : Inport  Port=2
  cfblk3 : Sqrt
  cfblk4 : Sqrt  Operator=rSqrt  AlgorithmType=Newton-Raphson
  cfblk5 : Sum  Inputs=+-
  cfblk6 : Sqrt
  cfblk2 : Outport
  cfblk8 : Outport  Port=2
  wires:
  cfblk6/1 -> cfblk3/1
  cfblk5/1 -> cfblk8/1
  cfblk7/1 -> cfblk4/1
  cfblk1/1 -> cfblk6/1, cfblk2/1
  cfblk3/1 -> cfblk5/1
  cfblk4/1 -> cfblk5/2

== system sampleModel1488/cfblk143/cfblk7 ==
  cfblk1 : Inport
  cfblk9 : Inport  Port=2
  cfblk10 : Inport  Port=3
  cfblk11 : Inport  Port=4
  cfblk12 : Inport  Port=5
  cfblk14 : Delay  SampleTime=1
  cfblk3 : DiscreteFir  SampleTime=1
  cfblk4 : Polyval  Coefs=[ +2.081618890e-019, -1.441693666e-014, +4.719686976e-010, -8.536869453e-006, +1.621573104e-001, -8.087801117e+001 ]
  cfblk5 : Math  Operator=10^u
  cfblk6 : Bias  Bias=[665883965.928379]  SaturateOnIntegerOverflow=off
  cfblk7 : Sin  TimeSource=Use external signal  SampleTime=0
  cfblk8 : Sin  TimeSource=Use external signal  SampleTime=0
  cfblk2 : Outport
  cfblk13 : Outport  Port=2
  wires:
  cfblk6/1 -> cfblk7/1
  cfblk9/1 -> cfblk8/1
  cfblk4/1 -> cfblk5/1
  cfblk11/1 -> cfblk2/1
  cfblk5/1 -> cfblk3/1
  cfblk10/1 -> cfblk4/1
  cfblk1/1 -> cfblk13/1
  cfblk7/1 -> cfblk14/1
  cfblk14/1 -> cfblk6/1
